simulink model "Total_AOA_and_Roll"  (R2018b)
settings: Solver=VariableStepAuto  StartTime=0.0  StopTime=10.0  RelTol=1e-3
libraries: simulink_extras x3
settings Model: Creator=auten  LastModifiedBy=auten

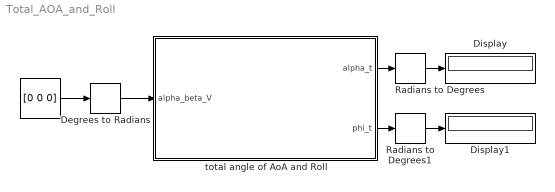
== system Total_AOA_and_Roll ==
  " " : Constant  Value=[0 0 0]  VectorParams1D=off  SampleTime=-1
  Degrees to Radians : simulink_extras/Transformations/Degrees to Radians
  Display : Display
  Display1 : Display
  Radians to Degrees : simulink_extras/Transformations/Radians to Degrees
  Radians to Degrees1 : simulink_extras/Transformations/Radians to Degrees
  total angle of AoA and Roll : Subsystem
  wires:
  " "/1 -> Degrees to Radians/1
  total angle of AoA and Roll/1(alpha_t) -> Radians to Degrees/1
  total angle of AoA and Roll/2(phi_t) -> Radians to Degrees1/1
  Degrees to Radians/1 -> total angle of AoA and Roll/1(alpha_beta_V)
  Radians to Degrees/1 -> Display/1
  Radians to Degrees1/1 -> Display1/1

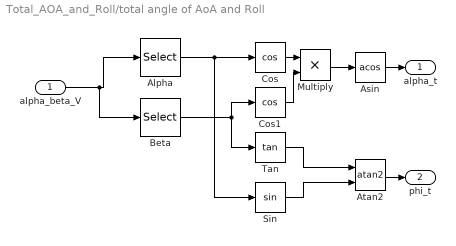
== system Total_AOA_and_Roll/total angle of AoA and Roll ==
  alpha_beta_V : Inport
  Alpha : Selector  InputPortWidth=3  IndexOptions=Index vector (dialog)  Indices=[1]  OutputSizes=1
  Asin : Trigonometry  Operator=acos
  Atan2 : Trigonometry  Operator=atan2
  Beta : Selector  InputPortWidth=3  IndexOptions=Index vector (dialog)  Indices=[2]  OutputSizes=1
  Cos : Trigonometry  Operator=cos
  Cos1 : Trigonometry  Operator=cos
  Multiply : Product
  Sin : Trigonometry
  Tan : Trigonometry  Operator=tan
  alpha_t : Outport
  phi_t : Outport  Port=2
  wires:
  Sin/1 -> Atan2/2
  Tan/1 -> Atan2/1
  Alpha/1 -> Sin/1, Cos/1
  Beta/1 -> Cos1/1, Tan/1
  Cos1/1 -> Multiply/2
  Multiply/1 -> Asin/1
  Cos/1 -> Multiply/1
  Atan2/1 -> phi_t/1
  Asin/1 -> alpha_t/1
  alpha_beta_V/1 -> Beta/1, Alpha/1
